simulink model "VHF_simulink_joystick"  (R2023a)
settings: Solver=VariableStepAuto  StartTime=0.0  StopTime=inf  RelTol=1e-3
model workspace (MAT data in the model file):
  SL_ROS_VariableLengthArrays_MaxSizes.CommonInfo.ArrayTruncateAction = 'EmitWarning'
  SL_ROS_VariableLengthArrays_MaxSizes.MsgTypeMap = containers.Map
  SL_ROS_VariableLengthArrays_MaxSizes.MsgTypeMap.serialization.keys = {'sensor_msgs/LaserScan'}
  SL_ROS_VariableLengthArrays_MaxSizes.MsgTypeMap.serialization.values{1}(1).PropertyName = 'intensities'
  SL_ROS_VariableLengthArrays_MaxSizes.MsgTypeMap.serialization.values{1}(1).DataType = 'single'
  SL_ROS_VariableLengthArrays_MaxSizes.MsgTypeMap.serialization.values{1}(1).MaxLength = 360
  SL_ROS_VariableLengthArrays_MaxSizes.MsgTypeMap.serialization.values{1}(2).PropertyName = 'ranges'
  SL_ROS_VariableLengthArrays_MaxSizes.MsgTypeMap.serialization.values{1}(2).DataType = 'single'
  SL_ROS_VariableLengthArrays_MaxSizes.MsgTypeMap.serialization.values{1}(2).MaxLength = 360
  SL_ROS_VariableLengthArrays_MaxSizes.MsgTypeMap.serialization.uniformity = 0
  SL_ROS_VariableLengthArrays_MaxSizes.MsgTypeMap.serialization.keyType = 'char'
  SL_ROS_VariableLengthArrays_MaxSizes.MsgTypeMap.serialization.valueType = 'any'
undefined symbols (not defined in the file): angular, linear
libraries: ros2lib x4, vrlib x1
settings Model: Creator=fede  LastModifiedBy=fede

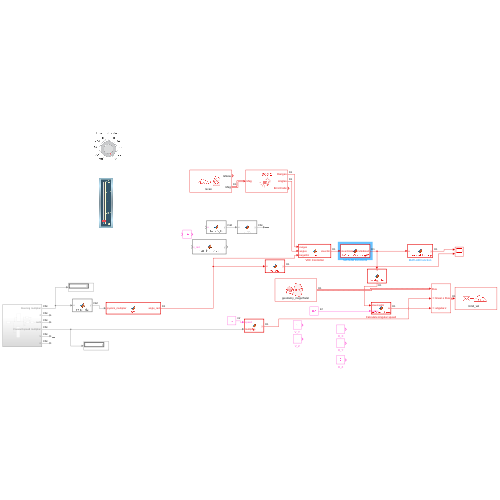
[thumbnail: Simulink's stored preview of the top-level diagram]
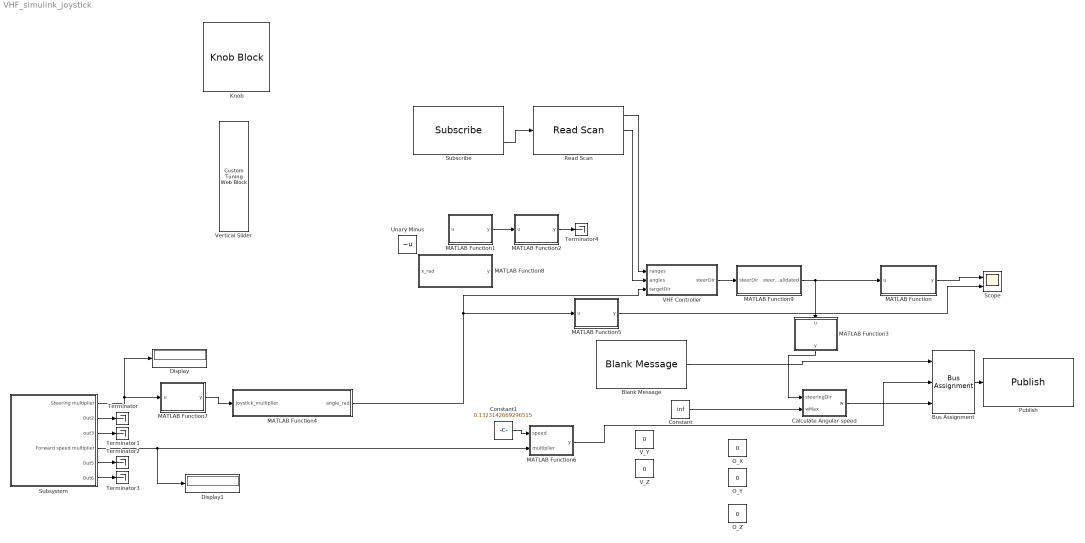
== system VHF_simulink_joystick ==
  Blank Message : ros2lib/Blank Message  messageClass=Message  entityType=geometry_msgs/Twist  messageType=geometry_msgs/Twist  SampleTime=0.01
  Bus Assignment : BusAssignment  AssignedSignals=linear.x,angular.z
  Calculate Angular speed : MATLAB Function  TreatAsAtomicUnit=on
  Constant : Constant  Value=inf
  Constant1 : Constant  Value=0.1323142669296515
  Display : Display
  Display1 : Display
  Knob : KnobBlock  ScaleMin=-90  ScaleMax=90
  MATLAB Function : MATLAB Function  TreatAsAtomicUnit=on
  MATLAB Function1 : MATLAB Function  TreatAsAtomicUnit=on
  MATLAB Function2 : MATLAB Function  TreatAsAtomicUnit=on
  MATLAB Function3 : MATLAB Function  TreatAsAtomicUnit=on
  MATLAB Function4 : MATLAB Function  TreatAsAtomicUnit=on  SystemSampleTime=0.01
  MATLAB Function5 : MATLAB Function  TreatAsAtomicUnit=on
  MATLAB Function6 : MATLAB Function  TreatAsAtomicUnit=on  SystemSampleTime=0.01
  MATLAB Function7 : MATLAB Function  TreatAsAtomicUnit=on
  MATLAB Function8 : MATLAB Function  TreatAsAtomicUnit=on
  MATLAB Function9 : MATLAB Function  TreatAsAtomicUnit=on
  O_X : Constant  Value=0
  O_Y : Constant  Value=0
  O_Z : Constant  Value=0
  Publish : ros2lib/Publish  topicSource=Select from ROS network  topic=/cmd_vel  messageType=geometry_msgs/Twist  QOSHistory=Keep last  QOSDepth=1  QOSReliability=Reliable  QOSDurability=Volatile
  Read Scan : ros2lib/Read Scan  MaximumArrayLength=100  ShowAnglesOutput=on  ShowIntensityOutput=off  ShowErrorCodeOutput=on  VariableSizeOutputs=off
  Scope : Scope  NumInputPorts=2
  Subscribe : ros2lib/Subscribe  topicSource=Select from ROS network  topic=/scan  messageType=sensor_msgs/LaserScan  sampleTime=0.01  QOSHistory=Keep last  QOSDepth=1  QOSReliability=Reliable  QOSDurability=Volatile
  Subsystem : Subsystem
  Terminator{,1..4} (5 alike) : Terminator
  Unary Minus : UnaryMinus
  VHF Controller : MATLAB Function  TreatAsAtomicUnit=on
  V_Y : Constant  Value=0
  V_Z : Constant  Value=0
  Vertical Slider : CustomTuningWebBlock  LabelPosition=Hide  ShowInitialText=on  Configuration="{\"components\":[{\"name\":\"LinearScaleComponent\",\"settings\":{\"bounds\":{\"max\":2,\"min\":0,\"tickInterval\":\"auto\"},\"internalTickHeightScaleFactor\":0.5,\"labelColor\":[255,255,200],\"labelFont\":{\"font\":\"Arial\",\"fontSize\":12},\"labelOffset\":0.05,\"labelTransparency\":1,\"needleImage\":{\"size\":[596,842],\"src\":\"data:image\\/svg+xml;base64,PD94bWwgdmVyc2lvbj0iMS4wIiBlbmNvZGluZz0idXRmLTgiPz4NCjwhLS0gR2VuZXJhdG9yOiBBZG9iZSBJbGx1c3RyYXRvciAyNS4wLjAsIFNWRyBFeHBvcnQgUGx1Zy1JbiAuIFNWRyBWZXJzaW9uOiA2LjAwIEJ1aWxkIDApICAtLT4NCjxzdmcgdmVyc2lvbj0iMS4xIg0KCSBpZD0ic3ZnOCIgeG1sbnM6Y2M9Imh0dHA6Ly9jcmVhdGl2ZWNvbW1vbnMub3JnL25zIyIgeG1sbnM6ZGM9Imh0dHA6Ly9wdXJsLm9yZy9kYy9lbGVtZW50cy8xLjEvIiB4bWxuczppbmtzY2FwZT0iaHR0cDovL3d3dy5pbmtzY2FwZS5vcmcvbmFtZXNw ...(+2420 chars)\",\"srcOrientation\":\"horizontal\"},\"needleOffset\":[0.0642123287671233,-0.8044596912521441],\"needleSize\":{\"height\":0.07668067226890757,\"width\":0.4337797619047619},\"position\":[0.03623949579831933,0.2829861111111111,0.6088789682539683,0.9196428571428571],\"referencePoint\":\"auto\",\"scaleColors\":[],\"scaleColorsSize\":0.2,\"scaleDirection\":\"BT\",\"showLabels\":1,\"showMinorTicks\":0,\"showSpanLine\":1,\"showTicks\":1,\"tickColor\":[252,252,197],\"tickTransparency\":1,\"valueBarColor\":[0,114,189],\"valueBarOffset\":-0.27,\"valueBarSize\":0.1,\"valueBarTransparency\":1}},{\"name\":\"BackgroundImageComponent\",\"settings\":{\"image\":{\"size\":[380,101],\"src\":\"data:image\\/svg+xml;base64,PHN2ZyB4bWxucz0iaHR0cDovL3d3dy53My5vcmcvMjAwMC9zdmciIHhtbG5zOnhsaW5rPSJodHRwOi8vd3d3LnczLm9yZy8xOTk5L3hsaW5rIiB2aWV3Qm94PSIwIDAgMzgwIDEwMSI+PGRlZnM+PHN0eWxlPi5jbHMtMXtmaWxsOiMwMDJiNDI7fS5jbHMtMntmaWxsOiM0MjcwODI7fS5jbHMtM3tmaWxsOnVybCgjcmFkaWFsLWdyYWRpZW50KTt9LmNscy00e2ZpbGw6I2M4YzhjODtzdHJva2U6IzAwMDt9PC9zdHlsZT48cmFkaWFsR3JhZGllbnQgaWQ9InJhZGlhbC1ncmFkaWVudCIgY3g9IjE5MCIgY3k9IjUwLjUiIHI9IjI2OS4yMSIgZ3JhZGllbnRVbml0cz0idXNlclNwYWNlT25Vc2UiPjxzdG9wIG9mZnNldD0iMC4wMSIgc3RvcC1jb2xvcj0iIzNlNGY1OCIvPjxzdG9wIG9mZnNldD0iMC4wNiIgc3RvcC1jb2xvcj0iIzQ0NTc2MSIvPjxzdG9wIG9mZnNldD0iMC4xNSIgc3RvcC1jb2xvcj0iIzU1NmE3NiIvPjxzdG9wIG9mZnNldD0iMC4yNSIgc3RvcC1jb2xvcj0iIzZkODg5NSIvPjxzdG9wIG9mZnNldD0iMC4zOCIgc3RvcC1jb2xvcj0iIzhmYjJjMyIvPjxzdG9wIG9mZnNldD0iMC41MiIgc3RvcC1jb2xvcj0iI2I2ZTRmYSIvPjxzdG9wIG9mZnNldD0iMSIgc3RvcC1jb2xvcj0iIzE1NDY1NyIvPjwvcmFkaWFsR3JhZGllbnQ+PC9kZWZzPjxnIGlkPSJmcmFtZSI+PGcgaWQ9IkxheWVyXzIiIGRhdGEtbmFtZT0iTGF5ZXIgMiI+PGcgaWQ9IkxheWVyXzEtMiIgZGF0YS1uYW1lPSJMYXllciAxLTIiPjxyZWN0IGlkPSJyZWN0MTAzNiIgY2xhc3M9ImNscy0xIiB4PSIxMSIgeT0iMTEiIHdpZHRoPSIzNTgiIGhlaWdodD0iNzkiLz48cGF0aCBpZD0icGF0aDEwMzgiIGNsYXNzPSJjbHMtMiIgZD0iTTgsOFY5M0gzNzJWOFpNMzY5LDkwSDExVjExSDM2OVoiLz48cGF0aCBpZD0icGF0aDEwNDAiIGNsYXNzPSJjbHMtMyIgZD0iTTAsMFYxMDFIMzgwVjBaTTM3Miw5M0g4VjhIMzcyWiIvPjwvZz48L2c+PC9nPjxnIGlkPSJ0cmFjayI+PHBhdGggaWQ9InJlY3QxNjExIiBjbGFzcz0iY2xzLTQiIGQ9Ik0zMy4zNywyNi41OUgzNDYuNjNjNCwwLDcuMjUsMi42LDcuMjUsNS44MWgwYzAsMy4yMS0zLjI1LDUuODItNy4yNSw1LjgySDMzLjM3Yy00LDAtNy4yNS0yLjYxLTcuMjUtNS44MmgwQzI2LjEyLDI5LjE5LDI5LjM3LDI2LjU5LDMzLjM3LDI2LjU5WiIvPjwvZz48L3N2Zz4=\",\"srcOrientation\":\"horizontal\"},\"position\":[0,0,1,1],\"scaleMode\":\"0\"}},{\"name\":\"ForegroundImageComponent\",\"settings\":{\"image\":{\"size\":[0,0],\"src\":\"default\",\"srcOrientation\":[]},\"isForeground\":1,\"position\":[0,0,1,1],\"scaleMode\":\"0\"}}],\"settings\":{\"BindingType\":\"param\",\"aspectRatio\":3.7777777777777777,\"backgroundColor\":[0,0,0,\"1\"],\"backgroundOffset\":0,\"backgroundOpacity\":1,\"fixedAspectRatio\":\"on\",\"foregroundColor\":[252,252,196],\"orientation\":\"vertical\",\"showBackgroundColor\":false,\"value\":0,\"version\":\"R2023a\"},\"type\":\"LinearGauge\"}"
  wires:
  Subscribe/2 -> Read Scan/1
  Read Scan/1 -> VHF Controller/1(ranges)
  Read Scan/2 -> VHF Controller/2(angles)
  MATLAB Function1/1(y) -> MATLAB Function2/1(u)
  VHF Controller/1(steerDir) -> MATLAB Function9/1(steerDir)
  MATLAB Function/1(y) -> Scope/1
  Blank Message/1 -> Bus Assignment/1
  Bus Assignment/1 -> Publish/1
  Subsystem/3(out3) -> Terminator1/1
  Subsystem/1(Steering multiplier) -> Display/1, MATLAB Function7/1(u)
  MATLAB Function5/1(y) -> Scope/2
  Subsystem/5(Out5) -> Terminator2/1
  Subsystem/6(Out6) -> Terminator3/1
  Subsystem/4(Forward speed multiplier) -> Display1/1, MATLAB Function6/2(multiplier)
  Subsystem/2(Out2) -> Terminator/1
  MATLAB Function6/1(y) -> Bus Assignment/2
  Constant1/1 -> MATLAB Function6/1(speed)
  MATLAB Function2/1(y) -> Terminator4/1
  MATLAB Function7/1(y) -> MATLAB Function4/1(joystick_multiplier)
  Calculate Angular speed/1(w) -> Bus Assignment/3
  MATLAB Function3/1(y) -> Calculate Angular speed/1(steeringDir)
  Constant/1 -> Calculate Angular speed/2(wMax)
  MATLAB Function4/1(angle_rad) -> MATLAB Function5/1(u), VHF Controller/3(targetDir)
  MATLAB Function9/1(steerDirValidated) -> MATLAB Function3/1(u), MATLAB Function/1(u)

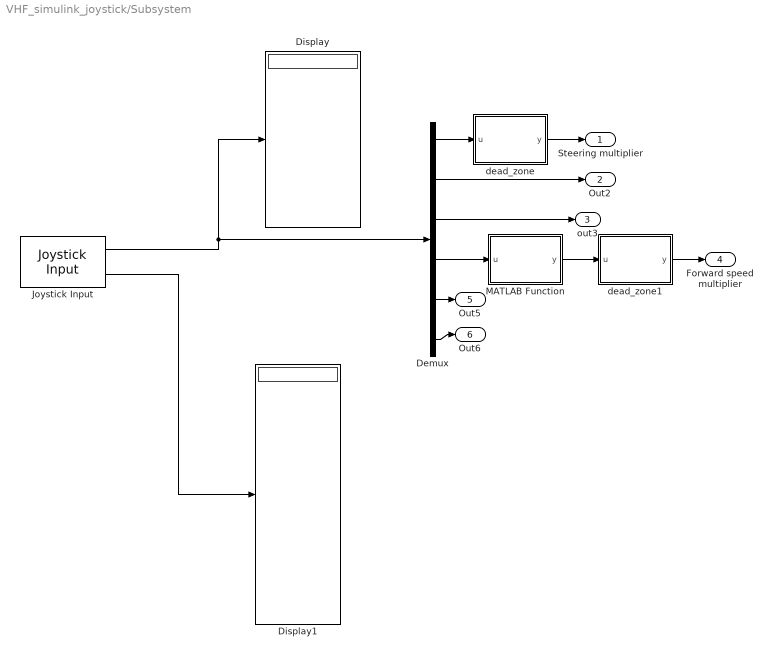
== system VHF_simulink_joystick/Subsystem ==
  Demux : Demux  Outputs=6
  Display : Display
  Display1 : Display
  Joystick Input : vrlib/Joystick Input  joyid=1  adjustports=on  forcefeed=off
  MATLAB Function : MATLAB Function  TreatAsAtomicUnit=on
  dead_zone : MATLAB Function  TreatAsAtomicUnit=on
  dead_zone1 : MATLAB Function  TreatAsAtomicUnit=on
  Steering multiplier : Outport
  Out2 : Outport  Port=2
  out3 : Outport  Port=3
  Forward speed multiplier : Outport  Port=4
  Out5 : Outport  Port=5
  Out6 : Outport  Port=6
  wires:
  Demux/2 -> Out2/1
  Demux/6 -> Out6/1
  Joystick Input/2 -> Display1/1
  Demux/5 -> Out5/1
  Joystick Input/1 -> Display/1, Demux/1
  Demux/3 -> out3/1
  MATLAB Function/1(y) -> dead_zone1/1(u)
  Demux/1 -> dead_zone/1(u)
  dead_zone/1(y) -> Steering multiplier/1
  Demux/4 -> MATLAB Function/1(u)
  dead_zone1/1(y) -> Forward speed multiplier/1

== matlab function VHF_simulink_joystick/Calculate Angular speed ==
  data: steeringDir input; w output; wMax input
function w = exampleHelperComputeAngularVelocity(steeringDir, wMax)
%EXAMPLEHELPERCOMPUTEANGULARVELOCITY Compute angular velocity
%   W = exampleHelperComputeAngularVelocity(STEERINGDIR)
%   returns the angular velocity W for a differential drive robot in radians
%   per second for a given steering direction STEERINGDIR in the robot's
%   coordinate frame in radians.
%
%   W = exampleHelperComputeAngularVelocity(STEERINGDIR, WMAX)
%   returns the angular velocity W for a differential drive robot in radians
%   per second for a given steering direction STEERINGDIR in the robot's
%   coordinate frame in radians and maximum angular velocity WMAX in
%   radians per second. The output angular velocity is saturated based on
%   the WMAX.
%
%   Example:
%       
%       w = exampleHelperComputeAngularVelocity(0.2, 1);

% Copyright 2015 The MathWorks, Inc.

%#codegen
%#ok<*EMCA>

% Allow variable input arguments
if nargin == 1   
    wMax = inf;
end

validateattributes(steeringDir, {'double'},{'real'},...
    'exampleHelperComputeAngularVelocity', 'STEERINGDIR', 1);
validateattributes(wMax, {'double'},{'real', 'positive'},...
    'exampleHelperComputeAngularVelocity', 'WMAX', 2);

% Computing in robot's coordinate frame
curPose = [0 0 0];

% The following computation is similar to robotics.PurePursuit
lookaheadPoint = [cos(steeringDir), sin(steeringDir)];
slope = atan2((lookaheadPoint(2) - curPose(2)), ...
    (lookaheadPoint(1) - curPose(1)));
alpha = angdiff(curPose(3), slope);

% Angular velocity command for a differential drive robot is
% equal to the desired curvature to be followed by the robot.

w = (2*sin(alpha));

% Pick a constant rotation when robot is facing in the opposite
% direction of the path
if abs(abs(alpha) - pi) < 1e-12
    w = sign(w)*1;
end

if abs(w) > wMax
    w = sign(w)*wMax;
end

end

== matlab function VHF_simulink_joystick/MATLAB Function9 ==
  data: steerDir input; steerDirValidated output
function steerDirValidated = checkValiditySteeringWheel(steerDir)

% if ~isnan(steerDir) % If steering direction is valid
% 	desiredV = 0.2;
% 	w = exampleHelperComputeAngularVelocity(steerDir,1);
% else % Stop and search for valid direction
% 	desiredV = 0.0;
% 	w = 0.5;
% end

if isnan(steerDir) % If steering direction is valid
    fprintf("%s\n","Invalid steeringDirection!")
end

steerDirValidated = steerDir;

== matlab function VHF_simulink_joystick/VHF Controller ==
  data: ranges input; steerDir output; angles input; targetDir input
function steerDir = fcn(ranges, angles, targetDir)

    vfh = controllerVFH;
    vfh.UseLidarScan = true;
    vfh.DistanceLimits = [0.05 1];
    vfh.RobotRadius = 0.1;
    vfh.MinTurningRadius = 0.2;
    vfh.SafetyDistance = 0.1;

    % Create a lidarScan object from the ranges and angles
    scan = lidarScan(ranges,angles);

    % plot(scan)

% Call VFH object to computer steering direction
    steerDir = vfh(scan, targetDir); 

    % h = figure;
    % set(h,'Position',[50 50 800 400])
    % show(vfh)

== matlab function VHF_simulink_joystick/MATLAB Function2 ==
  data: u input; y output
function y = to_rad(u)

y = deg2rad(u);

== matlab function VHF_simulink_joystick/MATLAB Function ==
  data: u input; y output
function y = from_rad_to_deg(u)

y = rad2deg(u);

== matlab function VHF_simulink_joystick/MATLAB Function3 ==
  data: u input; y output
function y = to_double(u)

y = double(u);

== matlab function VHF_simulink_joystick/MATLAB Function4 ==
  data: joystick_multiplier input; angle_rad output
function angle_rad = fcn(joystick_multiplier)

angle_rad = pi/4 * joystick_multiplier;

== matlab function VHF_simulink_joystick/MATLAB Function5 ==
  data: u input; y output
function y = to_deg(u)

y = rad2deg(u);

== matlab function VHF_simulink_joystick/Subsystem/MATLAB Function ==
  data: u input; y output
function y = fcn(u)
centered_value = u + 0.3616;

output_end = 1;
output_start = -1;
input_end = 0.7549;
input_start = -0.6384;

slope = (output_end - output_start) / (input_end - input_start);

y = -1*(output_start + slope * (centered_value - input_start));

== matlab function VHF_simulink_joystick/Subsystem/dead_zone ==
  data: u input; y output
function y = dead_zone(u)

if(abs(u) < 0.1)
    u=0;
end

y = u;

== matlab function VHF_simulink_joystick/Subsystem/dead_zone1 ==
  data: u input; y output
function y = dead_zone(u)

if(abs(u) < 0.1)
    u=0;
end

y = u;

== matlab function VHF_simulink_joystick/MATLAB Function6 ==
  data: speed input; y output; multiplier input
function y = fcn(speed, multiplier)

y = speed * multiplier;

== matlab function VHF_simulink_joystick/MATLAB Function7 ==
  data: u input; y output
function y = to_single(u)

y = single(u);

== matlab function VHF_simulink_joystick/MATLAB Function1 ==
  data: u input; y output
function y = to_single(u)

y = single(u);

== matlab function VHF_simulink_joystick/MATLAB Function8 ==
  data: x_rad input; y output
function y = map_into_0_2pi(x_rad)


y = wrapTo2Pi(x_rad);
